simulink model "communication_project2"  (R2021a)
settings: Solver=ode45  StartTime=0.0  StopTime=60  RelTol=1e-3  EnableMultiTasking=on
PreLoadFcn:
  | %%%%%%%%%%%%%%%%%%%%%%%%%%%%%%%%%%%%%%%%%%%%%%%%%%%%%%%%%%%%%%%%%%%%%%%%%%%
  | % check to see if Simulink library folder is missing from the MATLAB path %
  | %%%%%%%%%%%%%%%%%%%%%%%%%%%%%%%%%%%%%%%%%%%%%%%%%%%%%%%%%%%%%%%%%%%%%%%%%%%
  | if isempty(strfind(path, 'rtlsdr_book_library'))
  | 
  |     % create error window
  |     fig_error = figure(...
  |         'Name', 'Error: RTL-SDR Book Library',...
  |         'Toolbar','none',...
  |         'MenuBar','none',...
  |         'NumberTitle','off',...
  |         'Resize','off',...
  |         'WindowStyle','modal');
  |     fig_error.Position(3) = 600;
  |     fig_error.Position(4) = 150;
  |     fig_axes = axes(...
  |         'Parent',fig_error,...
  |         'Position',[0,0,1,1],...
  |         'visible','off');
  |     % error message
  |     t_title = text(.05,.8,...
  |         'MISSING DIRECTORIES',...
  |         'FontSize',11.5);
  |     t_body = text(.075,.6,...
  |         [{'Simulink cannot find the  \it{<root>}\rm / \it{rtlsdr\_book\_library}\rm  folder in the \it{MATLAB Path}\rm.'},...
  |         {'Please set the MATLAB path following the instructions given in Exercise 2.4.'}],...
  |         'FontSize',10.5);
  |     % buttons
  |     btn_path = uicontrol(...
  |         'Parent',fig_error,...
  |         'String','Set Path Now',...
  |         'FontSize',10,...
  |         'Callback', 'pathtool; close(fig_error);',...
  |         'Position', [fig_error.Position(3)/2-210, 30, 200, 30]);
  |     btn_abort = uicontrol(...
  |         'Parent',fig_error,...
  |         'String','No thanks',...
  |         'FontSize',10,...
  |         'Callback', 'close(fig_error); abort=1;',...
  |         'Position', [fig_error.Position(3)/2+10, 30, 200, 30]);
  | 
  |     % pause to allow user to interact with error box
  |     uiwait(fig_error);
  | 
  |     % abort simulation
  |     try
  |         if abort==1
  |             set_param(gcs, 'SimulationCommand', 'stop');
  |         end
  |     end
  | 
  |     % if user has set path, allow diagram to be updated
  |     if ~exist('abort','var')
  |         % create error window
  |         fig_update = figure(...
  |             'Name', 'Update Diagram',...
  |             'Toolbar','none',...
  |             'MenuBar','none',...
  |             'NumberTitle','off',...
  |             'Resize','off');
  |         fig_update.Position(3) = 400;
  |         fig_update.Position(4) = 120;
  |         fig_axes = axes(...
  |             'Parent',fig_update,...
  |             'Position',[0,0,1,1],...
  |             'visible','off');
  |         % instruction message
  |         t_body = text(.075,.7,...
  |             'Once you have set the path, update the block diagram',...
  |             'FontSize',10.5);
  |         % button
  |         btn_update = uicontrol(...
  |             'Parent',fig_update,...
  |             'String','Update Block Diagram',...
  |             'FontSize',10,...
  |             'Callback', 'set_param(gcs,''SimulationCommand'',''update''); close(gcf)',...
  |             'Position', [fig_update.Position(3)/2-100, 30, 200, 30]);
  |     end
  | 
  |     % clear error components
  |     clear('fig_error','fig_update','fig_axes','t_title','t_body','btn_path','btn_abort','btn_update','abort');
  | 
  | end
  | %%%%%%%%%%%%%%%%%%%%%%%%%%%%%%%%%%%%%%%%%%%%%%%%%%%%%%%%%%%%%%%%%%%%%%%%%%%
undefined symbols (not defined in the file): dfilt, fdesignblkfcn, gcbh, startfcn_spectrum_analyzer
libraries: dsparch4 x7, dspsrcs4 x2, dspvision x2, dspmlti4 x1, dspobslib x1
(part 1 of 2)
CloseFcn:
  | closefcn_model;
Description:
  | Software, Simulation Examples and Design Exercises Licence Agreement
  | 
  | This license agreement refers to the simulation examples, design exercises and files,
  | and associated software MATLAB and Simulink resources that accompany the book:
  | 
  |      Title: Software Defined Radio using MATLAB & Simulink and the RTL-SDR
  |      Published by Strathclyde Academic Media, 2015
  |      Authored by Robert W. Stewart, Kenneth W. Barlee, Dale S.W. Atkinson,
  |      and Louise H. Crockett
  | 
  | and made available as a download from, www.desktopSDR.com or variously acquired
  | by other means such as via USB storage, cloud storage, disk or any other electronic
  | or optical or magnetic storage mechanism. These files and associated software may
  | be used subject to the terms of agreement of the conditions below:
  | 
  |     Copyright © 2015 Robert W. Stewart, Kenneth W. Barlee, Dale S.W. Atkinson,
  |     and Louise H. Crockett
  |     All rights reserved.
  | 
  | Redistribution and use in source and binary forms, with or without modification, are
  | permitted provided that the following conditions are met:
  | 
  |    1.  Redistributions of source code must retain the above copyright notice, this list of
  |         conditions and the following disclaimer.
  | 
  |    2.  Redistributions in binary form must reproduce the above copyright notice, this
  |         list of conditions and the following disclaimer in the documentation and/or other
  |         materials provided with the distribution.
  | 
  |    3.  Neither the name of the copyright holder nor the names of its contributors may
  |         be used to endorse or promote products derived from this software without
  |         specific prior written permission.
  | 
  |    4.  In all cases, the software is, and all modifications and derivatives of the
  |         software shall be, licensed to you solely for use in conjunction with The
  |         MathWorks, Inc. products and service offerings.
  | 
  | THIS SOFTWARE IS PROVIDED BY THE COPYRIGHT HOLDERS AND CONTRIBUTORS
  | "AS IS" AND ANY EXPRESS OR IMPLIED WARRANTIES, INCLUDING, BUT NOT LIMITED
  | TO, THE IMPLIED WARRANTIES OF MERCHANTABILITY AND FITNESS FOR A
  | PARTICULAR PURPOSE ARE DISCLAIMED. IN NO EVENT SHALL THE COPYRIGHT
  | HOLDER OR CONTRIBUTORS BE LIABLE FOR ANY DIRECT, INDIRECT, INCIDENTAL,
  | SPECIAL, EXEMPLARY, OR CONSEQUENTIAL DAMAGES (INCLUDING, BUT NOT
  | LIMITED TO, PROCUREMENT OF SUBSTITUTE GOODS OR SERVICES; LOSS OF USE,
  | DATA, OR PROFITS; OR BUSINESS INTERRUPTION) HOWEVER CAUSED AND ON ANY
  | THEORY OF LIABILITY, WHETHER IN CONTRACT, STRICT LIABILITY, OR TORT
  | (INCLUDING NEGLIGENCE OR OTHERWISE) ARISING IN ANY WAY OUT OF THE USE
  | OF THIS SOFTWARE, EVEN IF ADVISED OF THE POSSIBILITY OF SUCH DAMAGE.
  | 
  | 
  | Audio Tracks used in Simulations Examples and Design Exercises
  | 
  | The music and vocal files used within the Examples files and software within the book
  | were variously written, arranged, performed, recorded and produced by Garrey Rice,
  | Adam Struth, Jamie Struth, Iain Thistlethwaite and also Marshall Craigmyle who
  | collectively, and individually where appropriate, assert and retain all of their copyright,
  | performance and artistic rights. Permission to use and reproduce this music is
  | granted for all purposes associated with MATLAB and Simulink software and the
  | simulation examples and design exercises files that accompany this book. Requests to
  | use the music for any other purpose should be directed to: info@desktopSDR.com.
  | For information on music track names, full credits, and links to the musicians please
  | refer to www.desktopSDR.com/more/audio.
settings Model: Creator=desktopSDR Team  LastModifiedBy=user
settings SolverCC: AlgebraicLoopSolver=TrustRegion
settings DataIOCC: SaveFormat=Array  SaveOutput=off  SignalLogging=off  SaveTime=off  ReturnWorkspaceOutputs=off
settings OptimizationCC: LifeSpan=inf
settings DebuggingCC: SolverPrmCheckMsg=warning  SFUnexpectedBacktrackingDiag=warning  SFNoUnconditionalDefaultTransitionDiag=warning  SFExecutionAtInitializationDiag=none  SFMachineParentedDataDiag=warning  ArithmeticOperatorsInVariantConditions=warning
settings HardwareCC: ProdBitPerPointer=32  ProdBitPerSizeT=32  ProdBitPerPtrDiffT=32  ProdLargestAtomicFloat=None  ProdIntDivRoundTo=Undefined  ProdEndianess=Unspecified  ProdWordSize=32  ProdHWDeviceType=32-bit Generic
settings ModelReferenceCC: PropagateSignalLabelsOutOfModel=off
settings SFSimCC: SimUseLocalCustomCode=off  CustomCodeUndefinedFunction=UseInterfaceOnly
settings RTWCC: RTWUseLocalCustomCode=off
settings CodeAppCC: StateflowObjectComments=on
settings GRTTargetCC: TargetLangStandard=C89/C90 (ANSI)
settings ConfigComp: CovMetricSettings=dw  CovSaveCumulativeToWorkspaceVar=on  CovSaveSingleToWorkspaceVar=on  CovExternalEMLEnable=off  CovSFcnEnable=off

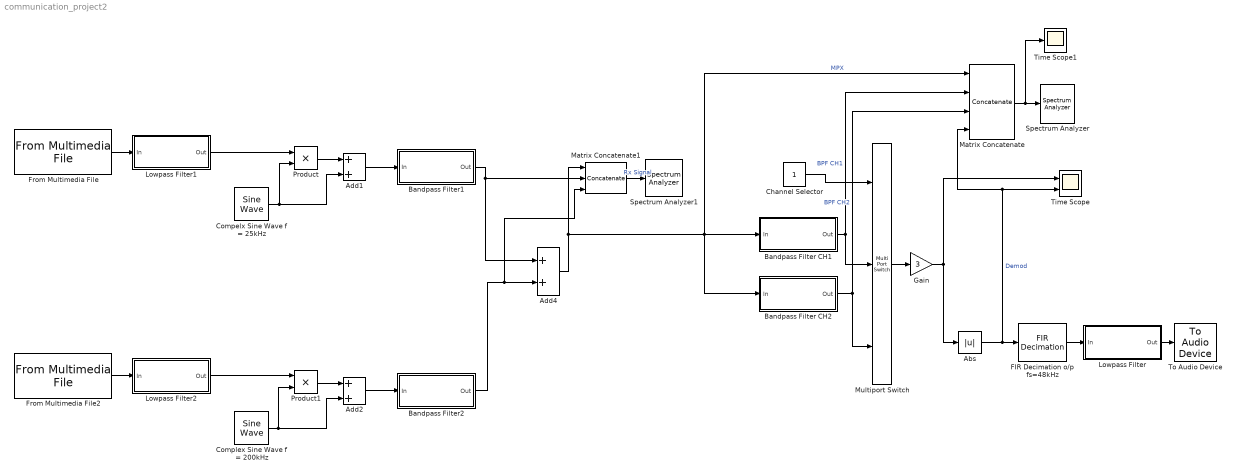
== system communication_project2 ==
  Abs : Abs
  Add1 : Sum
  Add2 : Sum
  Add4 : Sum
  Bandpass Filter CH1 : Subsystem  DialogController=fdesignblkfcn  InitFcn=fdesignblkfcn(gcbh, {'InitFcn'});  mask(Bandpass Filter){}
      mask help: Design a bandpass filter
      settings: CopyFcn=fdesignblkfcn(gcbh, {'CopyFcn'});
      mask Help: helpview(mapfilelocation('dsp'), 'dspbandpassfilter');
      mask Display: disp('Bandpass');
  Bandpass Filter CH2 : Subsystem  DialogController=fdesignblkfcn  InitFcn=fdesignblkfcn(gcbh, {'InitFcn'});  mask(Bandpass Filter){}
      mask help: Design a bandpass filter
      settings: CopyFcn=fdesignblkfcn(gcbh, {'CopyFcn'});
      mask Help: helpview(mapfilelocation('dsp'), 'dspbandpassfilter');
      mask Display: disp('Bandpass');
  Bandpass Filter1 : Subsystem  DialogController=fdesignblkfcn  InitFcn=fdesignblkfcn(gcbh, {'InitFcn'});  mask(Bandpass Filter){}
      mask help: Design a bandpass filter
      settings: CopyFcn=fdesignblkfcn(gcbh, {'CopyFcn'});
      mask Help: helpview(mapfilelocation('dsp'), 'dspbandpassfilter');
      mask Display: disp('Bandpass');
  Bandpass Filter2 : Subsystem  DialogController=fdesignblkfcn  InitFcn=fdesignblkfcn(gcbh, {'InitFcn'});  mask(Bandpass Filter){}
      mask help: Design a bandpass filter
      settings: CopyFcn=fdesignblkfcn(gcbh, {'CopyFcn'});
      mask Help: helpview(mapfilelocation('dsp'), 'dspbandpassfilter');
      mask Display: disp('Bandpass');
  Channel Selector : Constant
  Compelx Sine Wave f = 25kHz : dspsrcs4/Sine Wave  Amplitude=2  Frequency=25e3  Phase=0  SampleMode=Discrete  OutComplex=Complex  CompMethod=Trigonometric fcn  TableSize=Speed  SampleTime=1/48e3  SamplesPerFrame=600  ResetState=Restart at time zero  OutputFrames=on  dataType=double  wordLen=16  udDataType=sfix(16)  fracBitsMode=Best precision  numFracBits=15  OutDataTypeStr=double  LastOutDataTypeStr=double
  Complex Sine Wave f = 200kHz : dspsrcs4/Sine Wave  Amplitude=2  Frequency=200e3  Phase=0  SampleMode=Discrete  OutComplex=Complex  CompMethod=Trigonometric fcn  TableSize=Speed  SampleTime=1/48e3  SamplesPerFrame=600  ResetState=Restart at time zero  OutputFrames=on  dataType=double  wordLen=16  udDataType=sfix(16)  fracBitsMode=Best precision  numFracBits=15  OutDataTypeStr=double  LastOutDataTypeStr=double
  FIR Decimation o/p fs=48kHz : dspmlti4/FIR Decimation  FilterSource=Dialog parameters  h=firpm(100, [0 15e3 20e3 (240e3/2)]/(240e3/2), [1 1 0 0], [1 1], 20)  D=5  filtStruct=Direct form  FilterObject=Hm_firdecim  InputProcessing=Columns as channels (frame based)  framing=Allow multirate processing  inputOffset=0  outputBufInitCond=0  roundingMode=Floor  overflowMode=off  firstCoeffDataTypeStr=Inherit: Same word length as input  firstCoeffMin=[]  firstCoeffMax=[]  firstCoeffLastDataTypeStr=Inherit: Same word length as input  outputDataTypeStr=Inherit: Same as accumulator  outputMin=[]  outputMax=[]  outputLastDataTypeStr=Inherit: Same as accumulator
  From Multimedia File : dspvision/From Multimedia File  inputFilename=C:\Users\user\Desktop\Communication\audio_sources\music1_mono48kHz.wav  readRange=[1 Inf]  loop=on  numPlays=inf  outputStreams=Audio only  videoDataType=single  audioDataType=double  inheritSampleTime=on  userDefinedSampleTime=1/30  noAudioOutput=off  isIntensityVideo=off  fourcc=RGB  colorVideoFormat=Separate color signals  outputEOF=off  dataOrg=Column-major  audioFrameSize=600  computeAudioFrameSize=off  outSamplingMode=Frame based
  From Multimedia File2 : dspvision/From Multimedia File  inputFilename=C:\Users\user\Desktop\Communication\audio_sources\music1_mono48kHz.wav  readRange=[1 Inf]  loop=on  numPlays=inf  outputStreams=Audio only  videoDataType=single  audioDataType=double  inheritSampleTime=on  userDefinedSampleTime=1/30  noAudioOutput=off  isIntensityVideo=off  fourcc=RGB  colorVideoFormat=Separate color signals  outputEOF=off  dataOrg=Column-major  audioFrameSize=600  computeAudioFrameSize=off  outSamplingMode=Frame based
  Gain : Gain  Gain=3
  Lowpass Filter : Subsystem  DialogController=fdesignblkfcn  InitFcn=fdesignblkfcn(gcbh, {'InitFcn'});  mask(Lowpass Filter){}
      mask help: Design a lowpass filter
      settings: CopyFcn=fdesignblkfcn(gcbh, {'CopyFcn'});
      mask Help: helpview(mapfilelocation('dsp'), 'dsplowpassfilter');
      mask Display: disp('Lowpass')
  Lowpass Filter1 : Subsystem  DialogController=fdesignblkfcn  InitFcn=fdesignblkfcn(gcbh, {'InitFcn'});  mask(Lowpass Filter){}
      mask help: Design a lowpass filter
      settings: CopyFcn=fdesignblkfcn(gcbh, {'CopyFcn'});
      mask Help: helpview(mapfilelocation('dsp'), 'dsplowpassfilter');
      mask Display: disp('Lowpass')
  Lowpass Filter2 : Subsystem  DialogController=fdesignblkfcn  InitFcn=fdesignblkfcn(gcbh, {'InitFcn'});  mask(Lowpass Filter){}
      mask help: Design a lowpass filter
      settings: CopyFcn=fdesignblkfcn(gcbh, {'CopyFcn'});
      mask Help: helpview(mapfilelocation('dsp'), 'dsplowpassfilter');
      mask Display: disp('Lowpass')
  Matrix Concatenate : Concatenate  NumInputs=4  Mode=Multidimensional array  ConcatenateDimension=2
  Matrix Concatenate1 : Concatenate  NumInputs=3  Mode=Multidimensional array  ConcatenateDimension=2
  Multiport Switch : MultiPortSwitch  Inputs=2
  Product : Product
  Product1 : Product
  Spectrum Analyzer1 : SpectrumAnalyzer
  Spectrum Analyzer : SpectrumAnalyzer  StartFcn=startfcn_spectrum_analyzer;
  Time Scope : Scope  NumInputPorts=2
      settings: StartFcn=startfcn_time_scope;
  Time Scope1 : Scope
  To Audio Device : dspobslib/To Audio Device  deviceName=Default  inheritSampleRate=on  sampleRate=44100  deviceDatatype=Determine from input data type  autoBufferSize=on  bufferSize=4096  queueDuration=1.0  defaultOutputChannelMapping=on  outputChannelMapping=1  outputNumUnderrunSamples=off
      settings: SourceProductBaseCode=DS
  wires:
  Matrix Concatenate/1 -> Time Scope1/1, Spectrum Analyzer/1
  Lowpass Filter/1(Out) -> To Audio Device/1
  Channel Selector/1 -> Multiport Switch/1
  Bandpass Filter CH2/1(Out) -> Matrix Concatenate/3, Multiport Switch/3  "BPF CH2"
  FIR Decimation o/p fs=48kHz/1 -> Lowpass Filter/1(In)
  Bandpass Filter CH1/1(Out) -> Matrix Concatenate/2, Multiport Switch/2  "BPF CH1"
  Multiport Switch/1 -> Gain/1
  Abs/1 -> Matrix Concatenate/4, Time Scope/2, FIR Decimation o/p fs=48kHz/1  "Demod"
  Gain/1 -> Time Scope/1, Abs/1
  Matrix Concatenate1/1 -> Spectrum Analyzer1/1  "Rx Signal"
  Product/1 -> Add1/1
  Product1/1 -> Add2/1
  Complex Sine Wave f = 200kHz/1 -> Add2/2, Product1/2
  Add4/1 -> Bandpass Filter CH2/1(In), Matrix Concatenate/1, Bandpass Filter CH1/1(In), Matrix Concatenate1/1  "MPX"
  Bandpass Filter1/1(Out) -> Matrix Concatenate1/2, Add4/1
  Lowpass Filter1/1(Out) -> Product/1
  From Multimedia File/1 -> Lowpass Filter1/1(In)
  Add2/1 -> Bandpass Filter2/1(In)
  Bandpass Filter2/1(Out) -> Add4/2, Matrix Concatenate1/3
  From Multimedia File2/1 -> Lowpass Filter2/1(In)
  Add1/1 -> Bandpass Filter1/1(In)
  Compelx Sine Wave f = 25kHz/1 -> Product/2, Add1/2
  Lowpass Filter2/1(Out) -> Product1/1

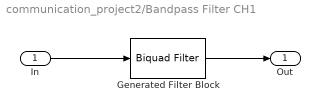
== system communication_project2/Bandpass Filter CH1 ==
  In : Inport
  Generated Filter Block : dsparch4/Biquad Filter  Tag=BlockMethodSubSystem  FilterSource=Dialog parameters  CoeffSource=Specify via dialog  FilterObject=dfilt.df2tsos([1 0.3 0.4],[1 0.1 0.2])  IIRFiltStruct=Direct form II  BiQuadCoeffs=[0.48710578309185842 0.020274699864626225 0.47606726400774318 1 -0.3200568934772296 0.9510875417757314;0.61694390478008665 -0.57271773922302893 0.60189559689807448 1 -0.68371663134321814 0.94964854256260212;0.84000114524790004 0.45824504577674063 0.021305946041866301 1 -0.48832315180999453 0.90165549195060035;0.0064548478739541466 0.011389175960501097 0.0049921122031908582 1 -0.72821163596699334 0.034855521810121665;0.77833495194845737 -0.20151009399259803 0.77832234721342286 1 -0.28213942704351702 0.99443660184789129;2 -1.5345249628396347 1.9997202303570027 1 -0.74285445349198365 0.99437926899504725;0.68303493454046227 0.074580654630850063 0.062904140898226851 1 -0.38577358709267945 0.9184389811629543;0.038054397531435698 -0.029838005454256376 0.0052742626653348402 1 -0.60016342729911176 0.91586675515872462;0.81687912100239568 -0.19207817940590149 0.81368134800883141 1 -0.29088293607338106 0.97858989499573013;2 -1.5735978982408823 1.9913568136029411 1 -0.7264857258290689 0.97824331105542206]  ScaleValues=[0.048249460042969664;1;1;1;1;1;1;1;1;1;10.550556890003632]  IC=0  ICnum=0  ICden=0  a0Flag=Warning  optimizeScaleValues=off  ScaleValueMode=Specify via input port (g)  InputProcessing=Columns as channels (frame based)  roundingMode=Floor  overflowMode=off  scaleValueFracLength=14  denProdOutputFracLength=30  denAccumFracLength=30  secondMemoryFracLength=15
  Out : Outport
  wires:
  Generated Filter Block/1 -> Out/1
  In/1 -> Generated Filter Block/1

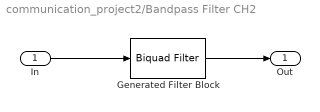
== system communication_project2/Bandpass Filter CH2 ==
  In : Inport
  Generated Filter Block : dsparch4/Biquad Filter  Tag=BlockMethodSubSystem  FilterSource=Dialog parameters  CoeffSource=Specify via dialog  FilterObject=dfilt.df2tsos([1 0.3 0.4],[1 0.1 0.2])  IIRFiltStruct=Direct form II  BiQuadCoeffs=[0.67338527760443312 -0.26671696059651728 0.6083593445883243 1 -0.19930278069396612 0.95848462181243144;0.5841637340870659 0.29230149777999481 0.56667307615551432 1 0.19906120642328817 0.9582828801664226;0.149036042446199 0.016946608863773197 0.010962149262872629 1 -0.052041795111932465 0.90786508164551083;0.020481807136560625 0.0032274650327607547 0.00012161868746611722 1 0.051117066171290415 0.9077685137822048;0.88089444047624554 -0.23157465446878642 0.88081993658726632 1 -0.23868838376901563 0.99490529520038307;2 0.52571694552187798 1.9997830967396211 1 0.23871035705725224 0.9948917802055679;0.75363304099796768 -0.50601088924497151 0.63927957482421738 1 -0.14123666236621696 0.929598737259827;0.057396929567661487 0.037309121966942291 0.051540971083893876 1 0.14053864118672826 0.92931947808271609;0.89113560972214434 -0.25188520382892204 0.89037379535859118 1 -0.22797195313135205 0.98116025020292619;2 0.56543358427809076 1.9989110580547198 1 0.22796205762099908 0.98109487138402474]  ScaleValues=[0.041299783151138178;1;1;1;1;1;1;1;1;1;10.556598798294175]  IC=0  ICnum=0  ICden=0  a0Flag=Warning  optimizeScaleValues=off  ScaleValueMode=Specify via input port (g)  InputProcessing=Columns as channels (frame based)  roundingMode=Floor  overflowMode=off  scaleValueFracLength=14  denProdOutputFracLength=30  denAccumFracLength=30  secondMemoryFracLength=15
  Out : Outport
  wires:
  Generated Filter Block/1 -> Out/1
  In/1 -> Generated Filter Block/1

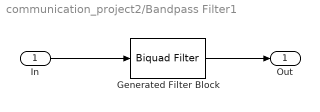
== system communication_project2/Bandpass Filter1 ==
  In : Inport
  Generated Filter Block : dsparch4/Biquad Filter  Tag=BlockMethodSubSystem  FilterSource=Dialog parameters  CoeffSource=Specify via dialog  FilterObject=BQF  IIRFiltStruct=Direct form II  BiQuadCoeffs=[1.1834868493177062 0 -1.1834868493177062 1 0.633896282140735012 0.951619406495656239;0.0692543543932287037 0 -0.0692543543932287037 1 -1.60982952387689426 0.934423128698709027;1.1285953560477322 0 -1.1285953560477322 1 0.600483602215051593 0.861529202773344327;0.110458490893193054 0 -0.110458490893193054 1 -1.53244525863600201 0.847171563419444218;1.07715639624040738 0 -1.07715639624040738 1 0.565972768964272177 0.779317579036856167;0.148379505949915391 0 -0.148379505949915391 1 -1.45629555464064531 0.765822935040603392;1.0282141462123362 0 -1.0282141462123362 1 0.530386013151578517 0.703957320390166896;0.99034592703271096 0 -0.99034592703271096 1 -1.38007999569957818 0.688867027166172208;0.306725009981402008 0 -0.306725009981402008 1 -1.31813615290074937 0.629608982061865663;0.225538342518794288 0 -0.225538342518794288 1 -1.30241414877044948 0.615038385254955244;1.54383081165229519 0 -1.54383081165229519 1 -1.23816245326644214 0.557474531461597977;0.503923924302058679 0 -0.503923924302058679 1 0.442892920946609037 0.55028238945025354;0.76815798215814135 0 -0.76815798215814135 1 0.403212362957007464 0.492436012164014003;0.297284361436536138 0 -0.297284361436536138 1 -1.15350404456053757 0.486516884001144401;0.99305123161776665 0 -0.99305123161776665 1 -1.08060145721815681 0.429910572680244851;0.455150104129165733 0 -0.455150104129165733 1 0.347817968325636051 0.421666776863955373;0.341240517160143808 0 -0.341240517160143808 1 -1.00093148433770152 0.372877253998972258;1.19350114295914023 0 -1.19350114295914023 1 -0.979627972194014207 0.358491983312663465;0.380687432991344943 0 -0.380687432991344943 1 0.24205047302353272 0.31328221127105399;0.415615053727591277 0 -0.415615053727591277 1 -0.886970535064595778 0.30024513420887039;1.06625050812643285 0 -1.06625050812643285 1 -0.807091299048777411 0.255784478237850998;0.725687171798046649 0 -0.725687171798046649 1 0.15691945640712518 0.246933067449949029;0.615065487793071575 0 -0.615065487793071575 1 0.0804649754094688835 0.200548708236959861;0.507586280582385863 0 -0.507586280582385863 1 -0.680048340944369611 0.196458458848929263;0.667712954011890791 0 -0.667712954011890791 1 -0.564600898975617937 0.155271367921023751;0.507860658403700982 0 -0.507860658403700982 1 -0.0305170791786006507 0.152241776429576231;0.517627204255238449 0 -0.517627204255238449 1 -0.13802391172100989 0.124067698601825954;0.5746870961187166 0 -0.5746870961187166 1 -0.168533250652107225 0.119072137358577898;0.538302993722273637 0 -0.538302993722273637 1 -0.350013500841746761 0.113806929530597192;0.487878522571731976 0 -0.487878522571731976 1 -0.235018867993249531 0.112440030105163472;0.614084238094004475 0 -0.614084238094004475 1 -0.0816612568808383205 0.136713331916494429;0.443847464031731698 0 -0.443847464031731698 1 -0.479109577200048098 0.133047192371139406;0.451954373109437979 0 -0.451954373109437979 1 0.0385128405245165131 0.179801275446719616;0.513984791639660599 0 -0.513984791639660599 1 0.0163955265958681783 0.170107945269130478;0.438726598187495265 0 -0.438726598187495265 1 -0.747027440089887751 0.22596004706839562;0.460981591028020943 0 -0.460981591028020943 1 0.119796760658597984 0.222964953472582217;0.439378719737350432 0 -0.439378719737350432 1 -0.861516879316862716 0.285491704635720989;0.401570126435592478 0 -0.401570126435592478 1 0.192159510951950246 0.272384861730488814;0.509773962697205762 0 -0.509773962697205762 1 0.273629436518011193 0.342363081288424131;0.485233175390528237 0 -0.485233175390528237 1 -0.934943115383428891 0.329519278195408494;0.432348432505243241 0 -0.432348432505243241 1 -1.04177329345855485 0.40147992016071854;0.5037847169367492 0 -0.5037847169367492 1 0.318878090793652147 0.388780941065237251;0.424355731455262897 0 -0.424355731455262897 1 -1.1177533338400174 0.458234249557397111;0.533412461236125179 0 -0.533412461236125179 1 0.375900366726550972 0.456188428369421028;0.4766354758708507 0 -0.4766354758708507 1 -1.20499211037261356 0.529007605325417019 ...(+6292 chars)]  ScaleValues=[0.0457559194366843405;1;1;1;1;1;1;1;1;1;1;1;1;1;1;1;1;1;1;1;1;1;1;1;1;1;1;1;1;1;1;1;1;1;1;1;1;1;1;1;1;1;1;1;1;1;1;1;1;1;1;1;1;1;1;1;1;1;1;1;1;1;1;1;1;1;1;1;1;1;1;1;1;1;1;1;1;1;1;1;1;1;1;1;1;1;1;1;1;1;1;1;1;1;1;1;1;1;1;1;1;1;1;1;1;1;1;1;1;1;1;1;1;1;1;1;1]  IC=0  ICnum=0  ICden=0  a0Flag=Warning  optimizeScaleValues=off  ScaleValueMode=Specify via input port (g)  InputProcessing=Columns as channels (frame based)  roundingMode=Floor  overflowMode=off  scaleValueFracLength=14  denProdOutputFracLength=30  denAccumFracLength=30  secondMemoryFracLength=15
  Out : Outport
  wires:
  Generated Filter Block/1 -> Out/1
  In/1 -> Generated Filter Block/1

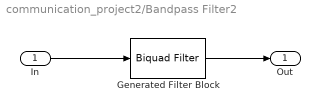
== system communication_project2/Bandpass Filter2 ==
  In : Inport
  Generated Filter Block : dsparch4/Biquad Filter  Tag=BlockMethodSubSystem  FilterSource=Dialog parameters  CoeffSource=Specify via dialog  FilterObject=BQF  IIRFiltStruct=Direct form II  BiQuadCoeffs=[1.1834868493177062 0 -1.1834868493177062 1 0.633896282140735012 0.951619406495656239;0.0692543543932287037 0 -0.0692543543932287037 1 -1.60982952387689426 0.934423128698709027;1.1285953560477322 0 -1.1285953560477322 1 0.600483602215051593 0.861529202773344327;0.110458490893193054 0 -0.110458490893193054 1 -1.53244525863600201 0.847171563419444218;1.07715639624040738 0 -1.07715639624040738 1 0.565972768964272177 0.779317579036856167;0.148379505949915391 0 -0.148379505949915391 1 -1.45629555464064531 0.765822935040603392;1.0282141462123362 0 -1.0282141462123362 1 0.530386013151578517 0.703957320390166896;0.99034592703271096 0 -0.99034592703271096 1 -1.38007999569957818 0.688867027166172208;0.306725009981402008 0 -0.306725009981402008 1 -1.31813615290074937 0.629608982061865663;0.225538342518794288 0 -0.225538342518794288 1 -1.30241414877044948 0.615038385254955244;1.54383081165229519 0 -1.54383081165229519 1 -1.23816245326644214 0.557474531461597977;0.503923924302058679 0 -0.503923924302058679 1 0.442892920946609037 0.55028238945025354;0.76815798215814135 0 -0.76815798215814135 1 0.403212362957007464 0.492436012164014003;0.297284361436536138 0 -0.297284361436536138 1 -1.15350404456053757 0.486516884001144401;0.99305123161776665 0 -0.99305123161776665 1 -1.08060145721815681 0.429910572680244851;0.455150104129165733 0 -0.455150104129165733 1 0.347817968325636051 0.421666776863955373;0.341240517160143808 0 -0.341240517160143808 1 -1.00093148433770152 0.372877253998972258;1.19350114295914023 0 -1.19350114295914023 1 -0.979627972194014207 0.358491983312663465;0.380687432991344943 0 -0.380687432991344943 1 0.24205047302353272 0.31328221127105399;0.415615053727591277 0 -0.415615053727591277 1 -0.886970535064595778 0.30024513420887039;1.06625050812643285 0 -1.06625050812643285 1 -0.807091299048777411 0.255784478237850998;0.725687171798046649 0 -0.725687171798046649 1 0.15691945640712518 0.246933067449949029;0.615065487793071575 0 -0.615065487793071575 1 0.0804649754094688835 0.200548708236959861;0.507586280582385863 0 -0.507586280582385863 1 -0.680048340944369611 0.196458458848929263;0.667712954011890791 0 -0.667712954011890791 1 -0.564600898975617937 0.155271367921023751;0.507860658403700982 0 -0.507860658403700982 1 -0.0305170791786006507 0.152241776429576231;0.517627204255238449 0 -0.517627204255238449 1 -0.13802391172100989 0.124067698601825954;0.5746870961187166 0 -0.5746870961187166 1 -0.168533250652107225 0.119072137358577898;0.538302993722273637 0 -0.538302993722273637 1 -0.350013500841746761 0.113806929530597192;0.487878522571731976 0 -0.487878522571731976 1 -0.235018867993249531 0.112440030105163472;0.614084238094004475 0 -0.614084238094004475 1 -0.0816612568808383205 0.136713331916494429;0.443847464031731698 0 -0.443847464031731698 1 -0.479109577200048098 0.133047192371139406;0.451954373109437979 0 -0.451954373109437979 1 0.0385128405245165131 0.179801275446719616;0.513984791639660599 0 -0.513984791639660599 1 0.0163955265958681783 0.170107945269130478;0.438726598187495265 0 -0.438726598187495265 1 -0.747027440089887751 0.22596004706839562;0.460981591028020943 0 -0.460981591028020943 1 0.119796760658597984 0.222964953472582217;0.439378719737350432 0 -0.439378719737350432 1 -0.861516879316862716 0.285491704635720989;0.401570126435592478 0 -0.401570126435592478 1 0.192159510951950246 0.272384861730488814;0.509773962697205762 0 -0.509773962697205762 1 0.273629436518011193 0.342363081288424131;0.485233175390528237 0 -0.485233175390528237 1 -0.934943115383428891 0.329519278195408494;0.432348432505243241 0 -0.432348432505243241 1 -1.04177329345855485 0.40147992016071854;0.5037847169367492 0 -0.5037847169367492 1 0.318878090793652147 0.388780941065237251;0.424355731455262897 0 -0.424355731455262897 1 -1.1177533338400174 0.458234249557397111;0.533412461236125179 0 -0.533412461236125179 1 0.375900366726550972 0.456188428369421028;0.4766354758708507 0 -0.4766354758708507 1 -1.20499211037261356 0.529007605325417019 ...(+6292 chars)]  ScaleValues=[0.0457559194366843405;1;1;1;1;1;1;1;1;1;1;1;1;1;1;1;1;1;1;1;1;1;1;1;1;1;1;1;1;1;1;1;1;1;1;1;1;1;1;1;1;1;1;1;1;1;1;1;1;1;1;1;1;1;1;1;1;1;1;1;1;1;1;1;1;1;1;1;1;1;1;1;1;1;1;1;1;1;1;1;1;1;1;1;1;1;1;1;1;1;1;1;1;1;1;1;1;1;1;1;1;1;1;1;1;1;1;1;1;1;1;1;1;1;1;1;1]  IC=0  ICnum=0  ICden=0  a0Flag=Warning  optimizeScaleValues=off  ScaleValueMode=Specify via input port (g)  InputProcessing=Columns as channels (frame based)  roundingMode=Floor  overflowMode=off  scaleValueFracLength=14  denProdOutputFracLength=30  denAccumFracLength=30  secondMemoryFracLength=15
  Out : Outport
  wires:
  In/1 -> Generated Filter Block/1
  Generated Filter Block/1 -> Out/1

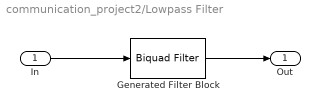
== system communication_project2/Lowpass Filter ==
  In : Inport
  Generated Filter Block : dsparch4/Biquad Filter  Tag=BlockMethodSubSystem  FilterSource=Dialog parameters  CoeffSource=Specify via dialog  FilterObject=dfilt.df2tsos([1 0.3 0.4],[1 0.1 0.2])  IIRFiltStruct=Direct form II  BiQuadCoeffs=[0.02505658453151734 0.050113169063034681 0.02505658453151734 1 -1.6618358052504689 0.92327518660477159;0.037716014607021689 0.075432029214043378 0.037716014607021689 1 -1.5666197180702381 0.81307974054400167;0.048494542600695072 0.096989085201390143 0.048494542600695072 1 -1.483833787366122 0.71726995848240305;0.057562689362794101 0.1151253787255882 0.057562689362794101 1 -1.4124095756411101 0.63460931673938947;0.065066669960849324 0.13013333992169865 0.065066669960849324 1 -1.3513355886493104 0.5639271931762575;0.071126049882347511 0.14225209976469502 0.071126049882347511 1 -1.2996951874675289 0.50416274358054824;0.075826965263644491 0.15165393052728898 0.075826965263644491 1 -1.2566848480829704 0.45438603384519421;0.079207708097762716 0.15841541619552543 0.079207708097762716 1 -1.2216205877683222 0.41380547733850032;0.081213644661423695 0.16242728932284739 0.081213644661423695 1 -1.1939377721788489 0.38176761165383055;0.08148106483340975 0.1629621296668195 0.08148106483340975 1 -1.1731876770814522 0.35775311943117882;0.076637308661870573 0.15327461732374115 0.076637308661870573 1 -1.1590329311748637 0.34137155424355531;0.047546496662289287 0.095092993324578573 0.047546496662289287 1 -1.1512431451247189 0.3323562819935113;0.04540058431321875 0.090801168626437501 0.04540058431321875 1 -1.1496915016555413 0.3305605345596806;0.045831247000341468 0.091662494000682937 0.045831247000341468 1 -1.1543527405881076 0.3359550778409825;0.046516257123944797 0.093032514247889594 0.046516257123944797 1 -1.1653027462029997 0.34862773420436555;0.047466760014933662 0.094933520029867324 0.047466760014933662 1 -1.1827197756415799 0.36878480413735909;0.048698191344618065 0.09739638268923613 0.048698191344618065 1 -1.2068872094697505 0.39675424952948513;0.050230457593599342 0.10046091518719868 0.050230457593599342 1 -1.2381975142107695 0.43299027958924174;0.052088101393404251 0.1041762027868085 0.052088101393404251 1 -1.2771568309371673 0.47807866131156473;0.054300385989436643 0.10860077197887329 0.054300385989436643 1 -1.3243891792379572 0.53274158481157419;0.056901193140924844 0.11380238628184969 0.056901193140924844 1 -1.3806386047689676 0.59784014872671409;0.059928568932260555 0.11985713786452111 0.059928568932260555 1 -1.4467665832625731 0.6743713558262725;0.063423665332839996 0.12684733066567999 0.063423665332839996 1 -1.5237404723519465 0.76345474808098879;0.023993836801624483 0.047987673603248966 0.023993836801624483 1 -1.612606599730263 0.86630126106162297;0.014199710532717848 0.028399421065435696 0.014199710532717848 1 -1.7144385404499303 0.98415336424243371;0.028453803345255303 0.056907606690510606 0.028453803345255303 1 -1.6368075882726612 0.89430953998294882;0.04083171761385794 0.08166343522771588 0.04083171761385794 1 -1.5448001049050344 0.78782747407497666;0.051459392354549008 0.10291878470909802 0.051459392354549008 1 -1.4649534370622368 0.69541935859814075;0.060531990296125222 0.12106398059225044 0.060531990296125222 1 -1.3962083671487442 0.61585934024476119;0.06815377125244737 0.13630754250489474 0.06815377125244737 1 -1.3375744913620335 0.54800120526008977;0.074455848419753085 0.14891169683950617 0.074455848419753085 1 -1.2881623105057174 0.49081551877004753;0.079552479596548167 0.15910495919309633 0.079552479596548167 1 -1.2471979145071224 0.44340661946156557;0.083510197687583193 0.16702039537516639 0.083510197687583193 1 -1.2140273488611264 0.40501767295371627;0.086395360489223874 0.17279072097844775 0.086395360489223874 1 -1.1881153515668013 0.37502921002970635;0.08825814050628647 0.17651628101257294 0.08825814050628647 1 -1.1690414739763555 0.35295463721924042;0.072653340568011524 0.14530668113602305 0.072653340568011524 1 -1.1564954726095342 0.33843490365490059;0.10631278825624907 0.21262557651249814 0.10631278825624907 1 -1.150273121708774 0.33123365486006179;0.09066349956390464 0.09066349956390464 0 1 -0.57474884697500372 0;0.045700079748393248 0.091400159496786496 0.045700079748393248 1 -1.1526025576110279 ...(+1162 chars)]  ScaleValues=[0.038531123333914737;1;1;1;1;1;1;1;1;1;1;1;1;1;1;1;1;1;1;1;1;1;1;1;1;1;1;1;1;1;1;1;1;1;1;1;1;1;1;1;1;1;1;1;1;1;1;1;1;1;1]  IC=0  ICnum=0  ICden=0  a0Flag=Warning  optimizeScaleValues=off  ScaleValueMode=Specify via input port (g)  InputProcessing=Columns as channels (frame based)  roundingMode=Floor  overflowMode=off  scaleValueFracLength=14  denProdOutputFracLength=30  denAccumFracLength=30  secondMemoryFracLength=15
  Out : Outport
  wires:
  Generated Filter Block/1 -> Out/1
  In/1 -> Generated Filter Block/1
